simulink subsystem "Pumpstation_Controller_Highpass"  (R2022b)
settings: Solver=VariableStepAuto  StartTime=0.0  StopTime=inf  RelTol=1e-3
model mask{Speedlimit_Upper=95, Speedlimit_Lower=65, Kp_ps1=0, Ki_ps1=0, TotalPumps_ps1=0, Kp_ps2=0, Ki_ps2=0, TotalPumps_ps2=0}
  mask prompts: Speedlimit_Upper "Upper limit on pump speed"; Speedlimit_Lower "Lower limit on pump speed"; Kp_ps1 "Kp for 1"; Ki_ps1 "Ki for 1"; TotalPumps_ps1 "Pumps availbale on 1"; Kp_ps2 "Kp for 2"; Ki_ps2 "Ki for 2"; TotalPumps_ps2 "Pumps available on 2"
libraries: dspfdesign x2, slpidlib x2
settings Model: DefaultTestHarness=Pumpstation_Controller_Highpass_Harness1  Creator=Fie  LastModifiedBy=pppc

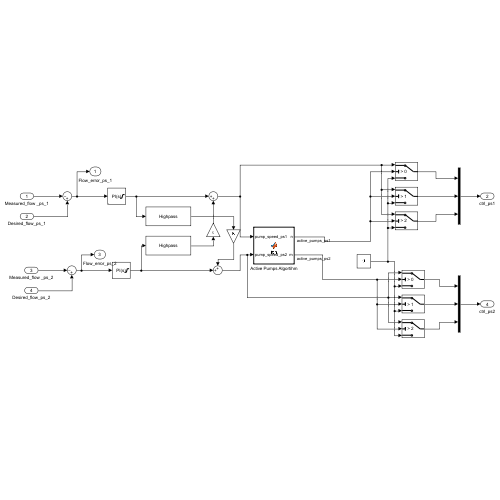
[thumbnail: Simulink's stored preview of the top-level diagram]
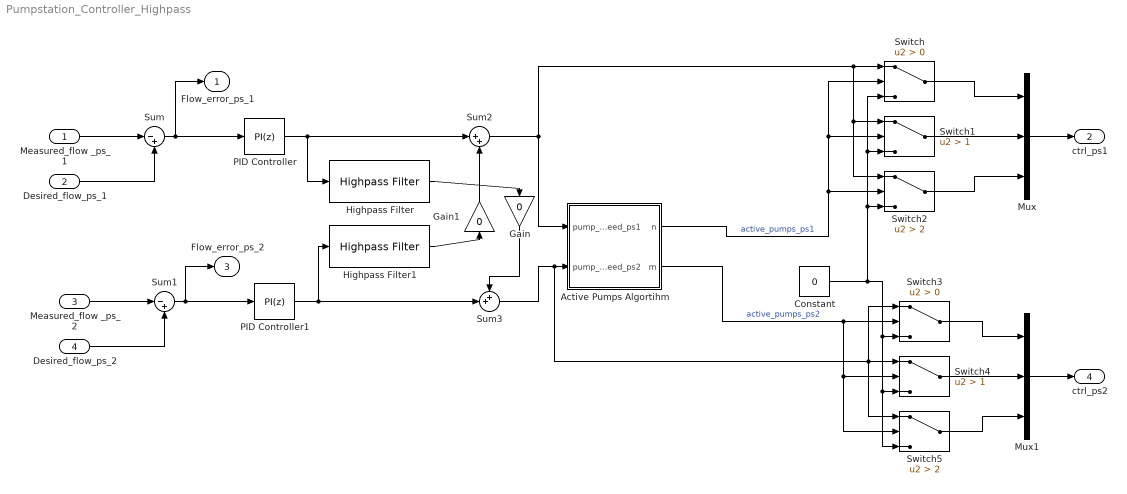
== system Pumpstation_Controller_Highpass ==
  Measured_flow _ps_1 : Inport
  Desired_flow_ps_1 : Inport  Port=2
  Measured_flow _ps_2 : Inport  Port=3
  Desired_flow_ps_2 : Inport  Port=4
  Active Pumps Algortihm : MATLAB Function  TreatAsAtomicUnit=on  SystemSampleTime=10
  Constant : Constant  Value=0
  Gain : Gain  Gain=0
  Gain1 : Gain  Gain=0
  Highpass Filter : dspfdesign/Highpass Filter  FilterType=FIR  DesignForMinimumOrder=on  FilterOrder=50  StopbandFrequency=0.05  PassbandFrequency=0.1  StopbandAttenuation=20  PassbandRipple=0.1  InheritSampleRate=off  SampleRate=1  SimulateUsing=Interpreted execution  roundingMode=Floor  coeffsDataTypeStr=fixdt(1,16)
  Highpass Filter1 : dspfdesign/Highpass Filter  FilterType=FIR  DesignForMinimumOrder=on  FilterOrder=50  StopbandFrequency=0.05  PassbandFrequency=0.1  StopbandAttenuation=80  PassbandRipple=0.1  InheritSampleRate=off  SampleRate=1  SimulateUsing=Interpreted execution  roundingMode=Floor  coeffsDataTypeStr=fixdt(1,16)
  Mux : Mux  Inputs=3
  Mux1 : Mux  Inputs=3
  PID Controller : slpidlib/PID Controller  Controller=PI  Form=Parallel  TimeDomain=Discrete-time  UseExternalTs=off  SampleTime=1  IntegratorMethod=Forward Euler  FilterMethod=Forward Euler  ControllerParametersSource=internal  P=Kp_ps1  I=Ki_ps1  UseKiTs=off  D=0  N=100  UseFilter=on  TunerSelectOption=Transfer Function Based (PID Tuner App)  InitialConditionSource=internal  InitialConditionForIntegrator=50  InitialConditionForFilter=0  DifferentiatorICPrevScaledInput=0  ExternalReset=none  TrackingMode=off  Kt=1  LimitOutput=on  SatLimitsSource=internal  UpperSaturationLimit=100  LowerSaturationLimit=0  LinearizeAsGain=on  AntiWindupMode=back-calculation  Kb=1  LimitIntegrator=off  UpperIntegratorSaturationLimit=inf  LowerIntegratorSaturationLimit=-inf  POutMin=[]  POutMax=[]  IOutMin=[]  IOutMax=[]  DOutMin=[]  DOutMax=[]  NOutMin=[]  NOutMax=[]  SumOutMin=[]  SumOutMax=[]  SaturationOutMin=[]  SaturationOutMax=[]  PParamMin=[]  PParamMax=[]  IParamMin=[]  IParamMax=[]  DParamMin=[]  DParamMax=[]  NParamMin=[]  NParamMax=[]  KbParamMin=[]  KbParamMax=[]  KtParamMin=[]  KtParamMax=[]  KbOutMin=[]  KbOutMax=[]  KtOutMin=[]  KtOutMax=[]  IntegratorOutMin=[]  IntegratorOutMax=[]  FilterOutMin=[]  FilterOutMax=[]  SumI1OutMin=[]  SumI1OutMax=[]  SumI2OutMin=[]  SumI2OutMax=[]  SumI3OutMin=[]  SumI3OutMax=[]  SumI4OutMin=[]  SumI4OutMax=[]  SumDOutMin=[]  SumDOutMax=[]  DifferentiatorOutMin=[]  DifferentiatorOutMax=[]  FilterDiffOutCoefMin=[]  FilterDiffOutCoefMax=[]  ReciprocalOutMin=[]  ReciprocalOutMax=[]  SumDenOutMin=[]  SumDenOutMax=[]  SumNumOutMin=[]  SumNumOutMax=[]  DivideOutMin=[]  DivideOutMax=[]  UdiffTsProdOutMin=[]  UdiffTsProdOutMax=[]  NTsProdOutMin=[]  NTsProdOutMax=[]  UintegralTsProdOutMin=[]  UintegralTsProdOutMax=[]  UngainTsProdOutMin=[]  UngainTsProdOutMax=[]  ClampingZeroOutDataTypeStr=Inherit: Inherit via back propagation  ClampingZeroOutMin=[]  ClampingZeroOutMax=[]  FilterDenConstantOutDataTypeStr=Inherit: Inherit via back propagation  FilterDenConstantOutMin=[]  FilterDenConstantOutMax=[]  PCopyOutDataTypeStr=Inherit: Inherit via back propagation  PCopyOutMin=[]  PCopyOutMax=[]  NCopyOutDataTypeStr=Inherit: Inherit via back propagation  NCopyOutMin=[]  NCopyOutMax=[]  IntegratorContinuousStateAttributes=''  IntegratorStateMustResolveToSignalObject=off  IntegratorRTWStateStorageClass=Auto  FilterContinuousStateAttributes=''  FilterStateMustResolveToSignalObject=off  FilterRTWStateStorageClass=Auto  ParallelPVariant=InternalParameters  IdealPVariant=Disabled  IVariant=InternalParameters  DVariant=Disabled  IntegratorVariant=Discrete  SatVariant=Enabled  AWVariant=BackCalculation  PCopyVariant=Disabled  TRVariant=Disabled  FdbkBlocksVariant=Forward  IdealPFdbkVariant=Disabled  SatFdbkVariant=Disabled  DerivativeFilterVariant=Disabled  NVariant=Disabled  NCopyVariant=Disabled_SignalSpec  FilterICVariant=Disabled  IntegratorICVariant=InternalICs  ExternalResetVariant=Disabled  TRSumVariant=Passthrough  SumFdbkVariant=Disabled  SumVariant=Sum_PI  TsampFilterVariant=InternalTs  TsampNgainVariant=Passthrough  TsampIntegralVariant=Passthrough  ExternalSaturationOutDataTypeStr=Inherit: Same as second input
  PID Controller1 : slpidlib/PID Controller  Controller=PI  Form=Parallel  TimeDomain=Discrete-time  UseExternalTs=off  SampleTime=1  IntegratorMethod=Forward Euler  FilterMethod=Forward Euler  ControllerParametersSource=internal  P=Kp_ps2  I=Ki_ps2  UseKiTs=off  D=0  N=100  UseFilter=on  TunerSelectOption=Transfer Function Based (PID Tuner App)  InitialConditionSource=internal  InitialConditionForIntegrator=50  InitialConditionForFilter=0  DifferentiatorICPrevScaledInput=0  ExternalReset=none  TrackingMode=off  Kt=1  LimitOutput=on  SatLimitsSource=internal  UpperSaturationLimit=100  LowerSaturationLimit=0  LinearizeAsGain=on  AntiWindupMode=back-calculation  Kb=1  LimitIntegrator=off  UpperIntegratorSaturationLimit=inf  LowerIntegratorSaturationLimit=-inf  POutMin=[]  POutMax=[]  IOutMin=[]  IOutMax=[]  DOutMin=[]  DOutMax=[]  NOutMin=[]  NOutMax=[]  SumOutMin=[]  SumOutMax=[]  SaturationOutMin=[]  SaturationOutMax=[]  PParamMin=[]  PParamMax=[]  IParamMin=[]  IParamMax=[]  DParamMin=[]  DParamMax=[]  NParamMin=[]  NParamMax=[]  KbParamMin=[]  KbParamMax=[]  KtParamMin=[]  KtParamMax=[]  KbOutMin=[]  KbOutMax=[]  KtOutMin=[]  KtOutMax=[]  IntegratorOutMin=[]  IntegratorOutMax=[]  FilterOutMin=[]  FilterOutMax=[]  SumI1OutMin=[]  SumI1OutMax=[]  SumI2OutMin=[]  SumI2OutMax=[]  SumI3OutMin=[]  SumI3OutMax=[]  SumI4OutMin=[]  SumI4OutMax=[]  SumDOutMin=[]  SumDOutMax=[]  DifferentiatorOutMin=[]  DifferentiatorOutMax=[]  FilterDiffOutCoefMin=[]  FilterDiffOutCoefMax=[]  ReciprocalOutMin=[]  ReciprocalOutMax=[]  SumDenOutMin=[]  SumDenOutMax=[]  SumNumOutMin=[]  SumNumOutMax=[]  DivideOutMin=[]  DivideOutMax=[]  UdiffTsProdOutMin=[]  UdiffTsProdOutMax=[]  NTsProdOutMin=[]  NTsProdOutMax=[]  UintegralTsProdOutMin=[]  UintegralTsProdOutMax=[]  UngainTsProdOutMin=[]  UngainTsProdOutMax=[]  ClampingZeroOutDataTypeStr=Inherit: Inherit via back propagation  ClampingZeroOutMin=[]  ClampingZeroOutMax=[]  FilterDenConstantOutDataTypeStr=Inherit: Inherit via back propagation  FilterDenConstantOutMin=[]  FilterDenConstantOutMax=[]  PCopyOutDataTypeStr=Inherit: Inherit via back propagation  PCopyOutMin=[]  PCopyOutMax=[]  NCopyOutDataTypeStr=Inherit: Inherit via back propagation  NCopyOutMin=[]  NCopyOutMax=[]  IntegratorContinuousStateAttributes=''  IntegratorStateMustResolveToSignalObject=off  IntegratorRTWStateStorageClass=Auto  FilterContinuousStateAttributes=''  FilterStateMustResolveToSignalObject=off  FilterRTWStateStorageClass=Auto  ParallelPVariant=InternalParameters  IdealPVariant=Disabled  IVariant=InternalParameters  DVariant=Disabled  IntegratorVariant=Discrete  SatVariant=Enabled  AWVariant=BackCalculation  PCopyVariant=Disabled  TRVariant=Disabled  FdbkBlocksVariant=Forward  IdealPFdbkVariant=Disabled  SatFdbkVariant=Disabled  DerivativeFilterVariant=Disabled  NVariant=Disabled  NCopyVariant=Disabled_SignalSpec  FilterICVariant=Disabled  IntegratorICVariant=InternalICs  ExternalResetVariant=Disabled  TRSumVariant=Passthrough  SumFdbkVariant=Disabled  SumVariant=Sum_PI  TsampFilterVariant=InternalTs  TsampNgainVariant=Passthrough  TsampIntegralVariant=Passthrough  ExternalSaturationOutDataTypeStr=Inherit: Same as second input
  Sum : Sum  Inputs=|-+
  Sum1 : Sum  Inputs=|-+
  Sum2 : Sum  Inputs=|++
  Sum3 : Sum  Inputs=++|
  Switch : Switch  Criteria=u2 > Threshold  SaturateOnIntegerOverflow=off  InputSameDT=off
  Switch1 : Switch  Criteria=u2 > Threshold  Threshold=1  SaturateOnIntegerOverflow=off  InputSameDT=off
  Switch2 : Switch  Criteria=u2 > Threshold  Threshold=2  SaturateOnIntegerOverflow=off  InputSameDT=off
  Switch3 : Switch  Criteria=u2 > Threshold  SaturateOnIntegerOverflow=off  InputSameDT=off
  Switch4 : Switch  Criteria=u2 > Threshold  Threshold=1  SaturateOnIntegerOverflow=off  InputSameDT=off
  Switch5 : Switch  Criteria=u2 > Threshold  Threshold=2  SaturateOnIntegerOverflow=off  InputSameDT=off
  Flow_error_ps_1 : Outport
  ctrl_ps1 : Outport  Port=2
  Flow_error_ps_2 : Outport  Port=3
  ctrl_ps2 : Outport  Port=4
  wires:
  Active Pumps Algortihm/1(n) -> Switch/2, Switch1/2, Switch2/2  "active_pumps_ps1"
  Switch1/1 -> Mux/2
  Switch2/1 -> Mux/3
  Desired_flow_ps_1/1 -> Sum/2
  Measured_flow _ps_1/1 -> Sum/1
  Sum/1 -> PID Controller/1, Flow_error_ps_1/1
  Switch/1 -> Mux/1
  PID Controller/1 -> Highpass Filter/1, Sum2/1
  Mux/1 -> ctrl_ps1/1
  Sum1/1 -> Flow_error_ps_2/1, PID Controller1/1
  Measured_flow _ps_2/1 -> Sum1/1
  Desired_flow_ps_2/1 -> Sum1/2
  Mux1/1 -> ctrl_ps2/1
  PID Controller1/1 -> Highpass Filter1/1, Sum3/2
  Switch3/1 -> Mux1/1
  Switch5/1 -> Mux1/3
  Switch4/1 -> Mux1/2
  Constant/1 -> Switch5/3, Switch4/3, Switch3/3, Switch2/3, Switch1/3, Switch/3
  Active Pumps Algortihm/2(m) -> Switch3/2, Switch5/2, Switch4/2  "active_pumps_ps2"
  Sum2/1 -> Active Pumps Algortihm/1(pump_speed_ps1), Switch1/1, Switch2/1, Switch/1
  Sum3/1 -> Switch3/1, Switch5/1, Switch4/1, Active Pumps Algortihm/2(pump_speed_ps2)
  Highpass Filter/1 -> Gain/1
  Highpass Filter1/1 -> Gain1/1
  Gain/1 -> Sum3/1
  Gain1/1 -> Sum2/2

== matlab function Pumpstation_Controller_Highpass/Active Pumps Algortihm ==
  data: pump_speed_ps1 input; n output; Speedlimit_Upper parameter; Speedlimit_Lower parameter; m output; TotalPumps_ps1 parameter; TotalPumps_ps2 parameter; pump_speed_ps2 input
function [n,m] = fcn(pump_speed_ps1, Speedlimit_Upper, Speedlimit_Lower, TotalPumps_ps1, TotalPumps_ps2, pump_speed_ps2)

persistent active_pumps_ps1
persistent active_pumps_ps2

if isempty(active_pumps_ps1)
    active_pumps_ps1 = 1;
end 
if isempty(active_pumps_ps2)
    active_pumps_ps2 = 1;
end 


if pump_speed_ps1 > Speedlimit_Upper 

    active_pumps_ps1 = min(active_pumps_ps1+1, TotalPumps_ps1);

elseif pump_speed_ps1 < Speedlimit_Lower

    active_pumps_ps1 = max(active_pumps_ps1-1, 1);

end

if pump_speed_ps2 > Speedlimit_Upper 

    active_pumps_ps2 = min(active_pumps_ps2+1, TotalPumps_ps2);

elseif pump_speed_ps2 < Speedlimit_Lower

    active_pumps_ps2 = max(active_pumps_ps2-1, 1);

end



n = active_pumps_ps1;
m = active_pumps_ps2;
